simulink model "Photovoltaic_Application_with_MPPT"  (R2017b)
settings: Solver=VariableStepDiscrete  StartTime=0.0  StopTime=0.1  MaxStep=5e-06  RelTol=1e-6
undefined symbols (not defined in the file): sigbuilder_block
libraries: powerlib x11, simulink x2, re_lib x1
settings Model: Creator=Damla  LastModifiedBy=dagac
settings SolverCC: AlgebraicLoopSolver=LineSearch

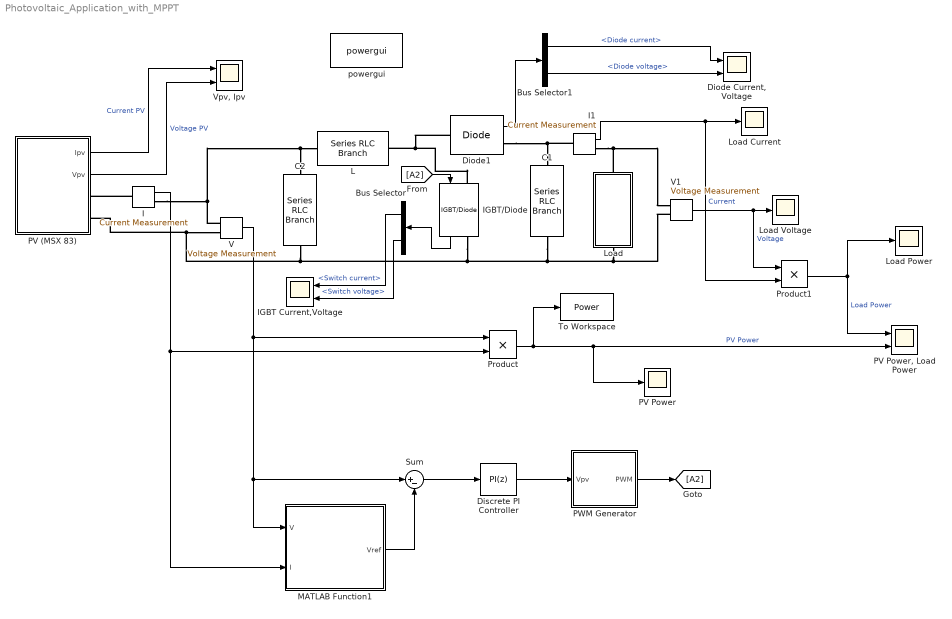
== system Photovoltaic_Application_with_MPPT ==
  Bus Selector : BusSelector  OutputSignals=Switch current,Switch voltage
  Bus Selector1 : BusSelector  OutputSignals=Diode current,Diode voltage
  "C1 " : powerlib/Elements/Series RLC Branch  LConnTagsString=__new0  RConnTagsString=__new0  BranchType=C  Resistance=10  Inductance=1e-3  SetiL0=off  InitialCurrent=0  Capacitance=220e-6  Setx0=off  InitialVoltage=0  Measurements=None
  "C2 " : powerlib/Elements/Series RLC Branch  LConnTagsString=__new0  RConnTagsString=__new0  BranchType=C  Resistance=10  Inductance=1e-3  SetiL0=off  InitialCurrent=0  Capacitance=250e-6  Setx0=off  InitialVoltage=0  Measurements=None
  "Diode Current, Voltage" : Scope  NumInputPorts=2
  Diode1 : powerlib/Power Electronics/Diode  Ron=1e-6  Lon=1e-6  Vf=0  IC=0  UseSnubber=0  Rs=1e-6  Cs=1e-6  Measurements=on
  Discrete PI Controller : simulink/Continuous/PID Controller  Controller=PI  TimeDomain=Discrete-time  SampleTime=-1  IntegratorMethod=Forward Euler  FilterMethod=Forward Euler  Form=Parallel  UseFilter=on  ControllerParametersSource=internal  P=0.0001  I=0.01  D=-1.08282271457395e-06  N=1.72043534996114  InitialConditionSource=internal  InitialConditionForIntegrator=0  InitialConditionForFilter=0  ExternalReset=none  LimitOutput=on  UpperSaturationLimit=0.95  LowerSaturationLimit=0  LinearizeAsGain=on  AntiWindupMode=clamping  Kb=1  TrackingMode=off  Kt=1  PParamMin=[]  PParamMax=[]  IParamMin=[]  IParamMax=[]  DParamMin=[]  DParamMax=[]  NParamMin=[]  NParamMax=[]  KbParamMin=[]  KbParamMax=[]  KtParamMin=[]  KtParamMax=[]  POutMin=[]  POutMax=[]  IOutMin=[]  IOutMax=[]  DOutMin=[]  DOutMax=[]  NOutMin=[]  NOutMax=[]  KbOutMin=[]  KbOutMax=[]  KtOutMin=[]  KtOutMax=[]  IntegratorOutMin=[]  IntegratorOutMax=[]  FilterOutMin=[]  FilterOutMax=[]  SumOutMin=[]  SumOutMax=[]  SumI1OutMin=[]  SumI1OutMax=[]  SumI2OutMin=[]  SumI2OutMax=[]  SumI3OutMin=[]  SumI3OutMax=[]  SumDOutMin=[]  SumDOutMax=[]  SaturationOutMin=[]  SaturationOutMax=[]  IntegratorContinuousStateAttributes=''  IntegratorStateMustResolveToSignalObject=off  IntegratorRTWStateStorageClass=Auto  FilterContinuousStateAttributes=''  FilterStateMustResolveToSignalObject=off  FilterRTWStateStorageClass=Auto  DifferentiatorICPrevScaledInput=0  DifferentiatorOutMin=[]  DifferentiatorOutMax=[]  InitialConditionSetting=State (most efficient)  FilterDiffOutCoefMin=[]  FilterDiffOutCoefMax=[]  SumDenOutMin=[]  SumDenOutMax=[]  SumNumOutMin=[]  SumNumOutMax=[]  ReciprocalOutMin=[]  ReciprocalOutMax=[]  DivideOutMin=[]  DivideOutMax=[]  TunerSelectOption=Transfer Function Based (PID Tuner App)
  I : powerlib/Measurements/Current Measurement  PhasorSimulation=off  OutputType=Complex  PSBequivalent=0
  I1 : powerlib/Measurements/Current Measurement  PhasorSimulation=off  OutputType=Complex  PSBequivalent=0
  IGBT Current,Voltage : Scope  NumInputPorts=2
  IGBT/Diode : powerlib/Power Electronics/IGBT//Diode  Ron=1e-6  Rs=1e-6  Cs=1e-6  Measurements=on
  L : powerlib/Elements/Series RLC Branch  LConnTagsString=__new0  RConnTagsString=__new0  BranchType=L  Resistance=10  Inductance=0.08e-3  SetiL0=off  InitialCurrent=0  Capacitance=1e-6  Setx0=off  InitialVoltage=0  Measurements=None
  Load : Subsystem
  Load Current : Scope
  Load Power : Scope
  Load Voltage : Scope
  MATLAB Function1 : MATLAB Function  TreatAsAtomicUnit=on
  PV (MSX 83) : Subsystem
  PV Power : Scope
  "PV Power, Load Power" : Scope  NumInputPorts=2
  PWM Generator : Subsystem
  Product : Product
  Product1 : Product
  Sum : Sum  Inputs=|+-
  To Workspace : ToWorkspace  VariableName=Power  SaveFormat=Timeseries  SampleTime=-1
  V : powerlib/Measurements/Voltage Measurement  PhasorSimulation=off  OutputType=Complex  PSBequivalent=0
  V1 : powerlib/Measurements/Voltage Measurement  PhasorSimulation=off  OutputType=Complex  PSBequivalent=0
  "Vpv, Ipv" : Scope  NumInputPorts=2
  powergui : powerlib/powergui  Priority=1  SimulationMode=Discrete  SampleTime=5e-07  frequency=60  Iterations=50  frequencyindice=0  Pbase=100e6  ErrMax=1e-4  UnitsV=kV  UnitsW=MW  buscounter=0  FunctionMessages=off  echomessages=off  EnableUseOfTLC=off  CurrentSourceSwitches=off  DisableSnubberDevices=off  DisableRonSwitches=off  DisableVfSwitches=off  DisplayEquations=off  SolverType=Tustin/Backward Euler (TBE)  Interpol=off  ExternalGateDelay=off  methode=off  Ts=100  x0status=blocks  SPID=on  SwTol=0  HookPort=off  RestoreLinks=warning  ResistiveCurrentMeasurement=off  Frange=[0:2:500]  Ylog=off  Xlog=on  ShowGrid=off  save=off  variable=ZData  structure=0  ZoomFFT=off  StartTime=0.0  cycles=1  DisplayStyle=1  fundamental=60  FreqAxis=off  MaxFrequency=1000  frequencyindicesteady=1  RmsSteady=1  display=off
  wires:
  PV (MSX 83)/2(Vpv) -> "Vpv, Ipv"/2  "Voltage PV"
  PWM Generator/1(PWM) -> [A2]
  Bus Selector/2 -> IGBT Current,Voltage/2  "<Switch voltage>"
  Diode1/1 -> Bus Selector1/1
  IGBT/Diode/1 -> Bus Selector/1
  Bus Selector1/2 -> "Diode Current, Voltage"/2  "<Diode voltage>"
  Bus Selector/1 -> IGBT Current,Voltage/1  "<Switch current>"
  I1/1 -> Product1/2, Load Current/1  "Current"
  Bus Selector1/1 -> "Diode Current, Voltage"/1  "<Diode current>"
  [A2] -> IGBT/Diode/1
  Product/1 -> To Workspace/1, PV Power/1, "PV Power, Load Power"/2  "PV Power"
  V1/1 -> Product1/1, Load Voltage/1  "Voltage"
  MATLAB Function1/1(Vref) -> Sum/2
  PV (MSX 83)/1(Ipv) -> "Vpv, Ipv"/1  "Current PV"
  I/1 -> MATLAB Function1/2(I), Product/2
  V/1 -> Product/1, MATLAB Function1/1(V), Sum/1
  Discrete PI Controller/1 -> PWM Generator/1(Vpv)
  Sum/1 -> Discrete PI Controller/1
  Product1/1 -> Load Power/1, "PV Power, Load Power"/1  "Load Power"
  connections:
  I1/LConn1 -- Diode1/RConn1 -- "C1 "/LConn1
  L/RConn1 -- IGBT/Diode/LConn1 -- Diode1/LConn1
  V/LConn1 -- L/LConn1 -- "C2 "/LConn1 -- I/RConn1
  I1/RConn1 -- V1/LConn1 -- Load/LConn1
  PV (MSX 83)/RConn2 -- IGBT/Diode/RConn1 -- V1/LConn2 -- Load/RConn1 -- "C1 "/RConn1 -- "C2 "/RConn1 -- V/LConn2
  I/LConn1 -- PV (MSX 83)/RConn1

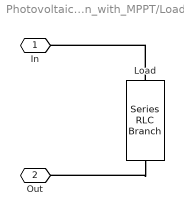
== system Photovoltaic_Application_with_MPPT/Load ==
  Load : powerlib/Elements/Series RLC Branch  LConnTagsString=__new0  RConnTagsString=__new0  BranchType=R  Resistance=14  Inductance=1e-3  SetiL0=off  InitialCurrent=0  Capacitance=1e-6  Setx0=off  InitialVoltage=0  Measurements=None
  In : PMIOPort  Port=1  Side=Left
  Out : PMIOPort  Port=2  Side=Right
  connections:
  Load/RConn1 -- Out/RConn1
  Load/LConn1 -- In/RConn1

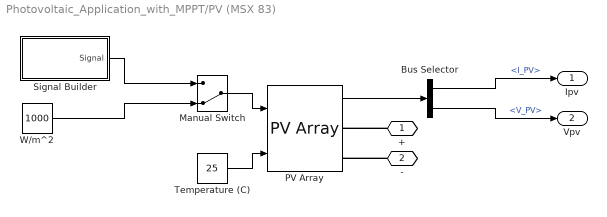
== system Photovoltaic_Application_with_MPPT/PV (MSX 83) ==
  Bus Selector : BusSelector  OutputSignals=I_PV,V_PV
  Manual Switch : ManualSwitch  CurrentSetting=0
  PV Array : re_lib/Solar/PV Array  Npar=1  Nser=4  PlotType=array @ 1000 W/m2 & specified temperatures  S_vec="[ 1000  500  100 ]"  Temp_C_vec="[ 25  ]"  ModuleName=User-defined  PlotWhenSelected=off  Pm=82.935  Ncell=36  Voc=21.2  Isc=5.27  Vm=17.1  Im=4.85  beta_Voc_pc=-0.38  alpha_Isc_pc=0.065  beta_Voc=-0.08056  alpha_Isc=0.0034255  IL=5.2836  I0=3.5018e-10  nI=0.97945  Rsh=115.354  Rs=0.29844  BAL=off  Tc=1e-6  Tfilter=5e-06
  Signal Builder : Subsystem  Tag=STV Subsys  LoadFcn=sigbuilder_block('load');  StartFcn=sigbuilder_block('start');  StopFcn=sigbuilder_block('stop');  ClipboardFcn=sigbuilder_block('clipboard');  mask(Sigbuilder block){tuvar=[0:10]}
      mask help: Simulink:masks:SigbuilderBlock_MD
      mask init:
      | if ~strcmp(get_param(bdroot(gcbh),'SimulationStatus'),'stopped') tuvar = sigbuilder_block('maskInit'); end
      settings: CopyFcn=sigbuilder_block('copy');  DeleteFcn=sigbuilder_block('delete');  ModelCloseFcn=sigbuilder_block('modelClose');  PreSaveFcn=sigbuilder_block('preSave');  PauseFcn=sigbuilder_block('pause');  ContinueFcn=sigbuilder_block('continue');  NameChangeFcn=sigbuilder_block('namechange');  OpenFcn=sigbuilder_block('open',[226.8 98.4 682.8 436.8 ]);  CloseFcn=sigbuilder_block('close');
      mask Display: plot(0, 0, 100, 100,[2, 2, 32, 32, 2], [68, 8, 8, 68, 68],[32, 2], [38, 38], [32, 19, 2],[53, 60, 44], [32, 17, 17, 2],[16, 16, 31, 31]);txt = getActiveGroup(gcbh);text(2, 100, txt,'verticalAlignment', 'top');
  Temperature (C) : Constant  Value=25
  W/m^2 : Constant  Value=1000
  + : PMIOPort  Port=1  Side=Right
  - : PMIOPort  Port=2  Side=Right
  Ipv : Outport
  Vpv : Outport  Port=2
  wires:
  Temperature (C)/1 -> PV Array/2
  Bus Selector/1 -> Ipv/1  "<I_PV>"
  Bus Selector/2 -> Vpv/1  "<V_PV>"
  PV Array/1 -> Bus Selector/1
  Signal Builder/1(Signal) -> Manual Switch/1
  W/m^2/1 -> Manual Switch/2
  Manual Switch/1 -> PV Array/1
  connections:
  -/RConn1 -- PV Array/RConn2
  +/RConn1 -- PV Array/RConn1

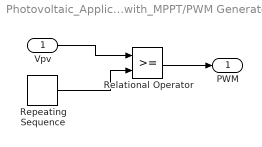
== system Photovoltaic_Application_with_MPPT/PWM Generator ==
  Vpv : Inport
  Relational Operator : RelationalOperator  OutDataTypeStr=boolean  RndMeth=Simplest
  Repeating Sequence : simulink/Sources/Repeating Sequence  rep_seq_t=[0 1/5000]  rep_seq_y=[0 1]
  PWM : Outport
  wires:
  Repeating Sequence/1 -> Relational Operator/2
  Relational Operator/1 -> PWM/1
  Vpv/1 -> Relational Operator/1

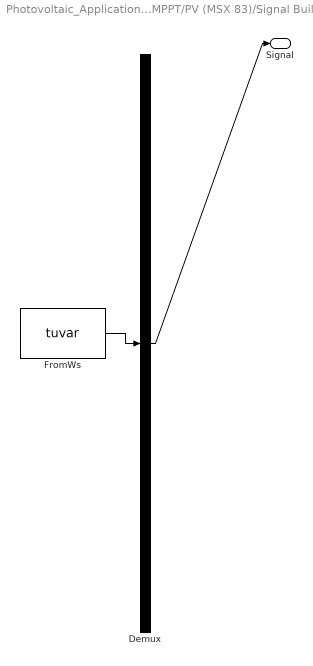
== system Photovoltaic_Application_with_MPPT/PV (MSX 83)/Signal Builder ==
  Demux : Demux  Tag=STV Demux  Outputs=1
  FromWs : FromWorkspace  Tag=STV FromWs  VariableName=tuvar  SampleTime=0
      SigBuilderData=|
      | common.afterFinalStr = 'Extrapolate'
      | common.sampleTime = 0
      | dataSet.timeRange = [0 10]
      | dataSet.name = 'Group 1'
      | sbobj.Groups.Name = 'Group 1'
      | sbobj.Groups.Signals.Name = 'Signal'
      | sbobj.Groups.Signals.XData = [0 0.03 0.04 0.06 0.06 10]
      | sbobj.Groups.Signals.YData = [1000 1000 600 600 400 0]
  Signal : Outport  Tag=STV Outport
  wires:
  FromWs/1 -> Demux/1
  Demux/1 -> Signal/1

== matlab function Photovoltaic_Application_with_MPPT/MATLAB Function1 ==
  data: V input; Vref output; I input
function Vref = MPPT(V,I)
Vrefmax = 75.24;
Vrefmin = 21.2;
Vrefinit = 61.56;
deltaVref = 0.74;
persistent Vold Pold Vrefold;
if isempty(Vold)
    Vold = 0;
    Pold = 0;
    Vrefold = Vrefinit;
end
P = V*I; dV = V-Vold; dP = P-Pold;
if dP ~= 0
    if dP < 0
        if dV < 0
            Vref = Vrefold + deltaVref;
        else
            Vref = Vrefold - deltaVref;
        end
    else
        if dV < 0
            Vref = Vrefold - deltaVref;
        else
            Vref = Vrefold + deltaVref;
        end
    end
else
    Vref = Vrefold;
end
if Vref >= Vrefmax || Vref <= Vrefmin
    Vref = Vrefold;
end
Vrefold = Vref; Vold = V; Pold = P;
